simulink model "Legobilen"  (R2024a)
settings: Solver=VariableStepAuto  StartTime=0.0  StopTime=10.0  RelTol=1e-3
values from neighbouring files (symbols this model uses):
  Acl = A - (B*K)    [Bilvariabler.m]
  Bcl = K0*B    [Bilvariabler.m]
  C = [k2 0]    [Bilvariabler.m]
settings Model: Creator=jesperbertelsen  LastModifiedBy=jesperbertelsen

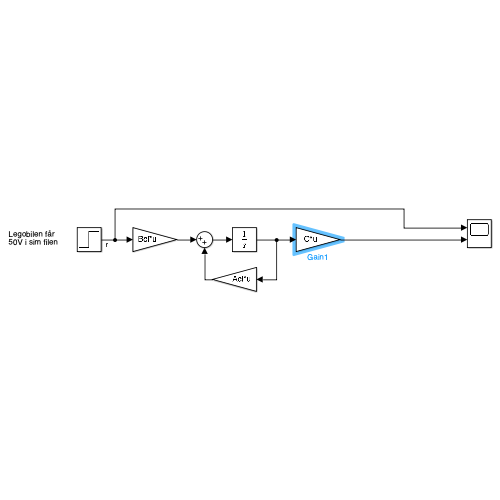
[thumbnail: Simulink's stored preview of the top-level diagram]
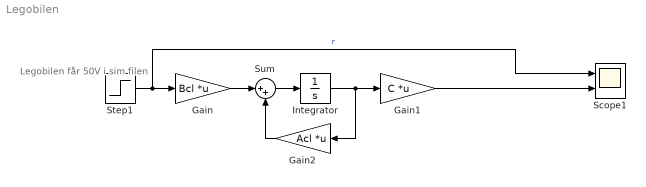
== system Legobilen ==
  note: Legobilen får 50V i sim filen
  Gain : Gain  Gain=Bcl  Multiplication=Matrix(K*u)
  Gain1 : Gain  Gain=C  Multiplication=Matrix(K*u)
  Gain2 : Gain  Gain=Acl  Multiplication=Matrix(K*u)
  Integrator : Integrator
  Scope1 : Scope  NumInputPorts=2
  Step1 : Step  After=50  SampleTime=0
  Sum : Sum  Inputs=|++
  wires:
  Step1/1 -> Gain/1, Scope1/1  "r"
  Integrator/1 -> Gain2/1, Gain1/1
  Gain1/1 -> Scope1/2
  Gain/1 -> Sum/1
  Sum/1 -> Integrator/1
  Gain2/1 -> Sum/2
